simulink model "radar_lidar_road_curve"  (R2021b)
settings: Solver=FixedStepDiscrete  StartTime=0.0  StopTime=10.0  RelTol=1e-3
model workspace (MAT data in the model file):
  firstWarning = 1
  originalScenarioChecksum = '173E6664BED95618E8BCACADB1E8F97C'
libraries: drivingscenarioandsensors x3
settings Model: Creator=ghisl  LastModifiedBy=ghisl

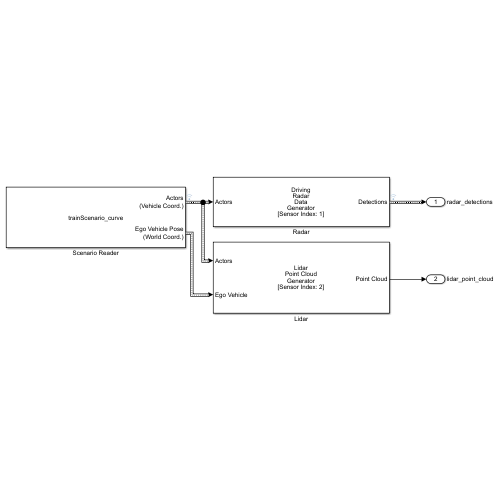
[thumbnail: Simulink's stored preview of the top-level diagram]
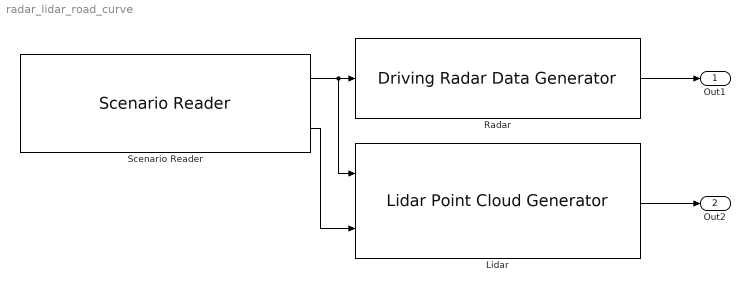
== system radar_lidar_road_curve ==
  Lidar : drivingscenarioandsensors/Lidar Point Cloud Generator  SensorIndex=2  UpdateInterval=0.1  SensorLocation=[0.05 0]  Height=1.6  Yaw=0  Pitch=0  Roll=0  DetectionCoordinates=Ego Cartesian  HasEgoVehicle=on  EgoVehicleActorID=2  HasRoadsInputPort=on  ActorProfilesSource=From Scenario Reader block  ActorProfilesVariableName=actor_profiles  MaxRange=120  RangeAccuracy=0.002  AzimuthResolution=0.16  ElevationResolution=1.25  AzimuthLimits=[-180 180]  ElevationLimits=[-20 20]  HasNoise=on
      settings: SourceProductBaseCode=DR
  Radar : drivingscenarioandsensors/Driving Radar Data Generator  SensorIndex=1  UpdateRate=10  MountingLocation=[1 0 0.2]  MountingAngles=[0 0 0]  HasElevation=off  HasRangeRate=on  HasNoise=on  HasFalseAlarms=on  HasOcclusion=on  MaxNumReportsSource=Property  MaxNumReports=50  TargetReportFormat=Detections  DetectionCoordinates=Body  TrackCoordinates=Body  BusNameSource=Auto  BusName=BusDrivingRadarDataGenerator  AzimuthResolution=4  ElevationResolution=5  RangeResolution=2.5  RangeRateResolution=0.5  AzimuthBiasFraction=0.1  ElevationBiasFraction=0.1  RangeBiasFraction=0.05  RangeRateBiasFraction=0.05  FieldOfView=[20 5]  RangeLimits=[0 100]  RangeRateLimits=[-100 100]  DetectionProbability=0.9  FalseAlarmRate=1e-06  ReferenceRange=100  ReferenceRCS=0  CenterFrequency=77000000000  FilterInitializationFcn=initcvekf  ConfirmationThreshold=[2 3]  DeletionThreshold=[5 5]  InitialSeedSource=Repeatable  InitialSeed=0  UsedSeed=0  ProfilesSource=Parameters  ProfilesParameters=driving.internal.ActorProfilesRadarParameters  ProfilesExpression=[struct('ActorID',1,'ClassID',7,'Length',20,'Width',2.8,'Height',4,'OriginOffset',[-9 0 0],'MeshVertices',[19 -1.4 4;19 1.4 4;-1 1.4 4;-1 -1.4 4;19 -1.4 0;19 1.4 0;-1 1.4 0;-1 -1.4 0],'MeshFaces',[6 2 1;1 5 6;8 4 3;3 7 8;6 7 3;3 2 6;5 1 4;4 8 5;4 1 2;2 3 4;7 6 5;5 8 7],'RCSPattern',[10 10;10 10],'RCSAzimuthAngles',[-180 180],'RCSElevationAngles',[-90 90]); struct('ActorID',2,'ClassID',8,'Length',2,'Width',0.6,'Height',1,'OriginOffset',[0 0 0],'MeshVertices',[1 0.3 0.612456747404844;1 -0.3 0.612456747404844;1 -0.3 0.224913494809689;1 0.3 0.224913494809689;1 0.3 0.612456747404844;0.5 0.3 0.709342560553633;0.5 -0.3 0.709342560553633;1 -0.3 0.612456747404844;0.2 0.24 1;-0.4 0.24 1;-0.4 -0.24 1;0.2 -0.24 1;-0.7 0.3 0.709342560553633;-1 0.3 0.612456747404844;-1 -0.3 0.612456747404844;-0.7 -0.3 0.709342560553633;1 0.3 0.612456747404844;1 0.3 0.224913494809689;0.5 0.3 0.224913494809689;0.5 0.3 0.709342560553633;0.5 0.3 0.709342560553633;0.5 0.3 0.224913494809689;-0.7 0.3 0.224913494809689;-0.7 0.3 0.709342560553633;-0.7 0.3 0.709342560553633;-0.7 0.3 0.224913494809689;-1 0.3 0.253979238754325;-1 0.3 0.612456747404844;0.5 0.3 0.709342560553633;-0.7 0.3 0.709342560553633;-0.4 0.24 1;0.2 0.24 1;1 -0.3 0.612456747404844;1 -0.3 0.224913494809689;0.5 -0.3 0.224913494809689;0.5 -0.3 0.709342560553633;0.5 -0.3 0.709342560553633;0.5 -0.3 0.224913494809689;-0.7 -0.3 0.224913494809689;-0.7 -0.3 0.709342560553633;-0.7 -0.3 0.709342560553633;-0.7 -0.3 0.224913494809689;-1 -0.3 0.253979238754325;-1 -0.3 0.612456747404844;0.5 -0.3 0.709342560553633;-0.7 -0.3 0.709342560553633;-0.4 -0.24 1;0.2 -0.24 1;-0.7 0.3 0.709342560553633;-0.7 -0.3 0.709342560553633;-0.4 -0.24 1;-0.4 0.24 1;0.5 -0.3 0.709342560553633;0.2 -0.24 1;0.2 0.24 1;0.5 0.3 0.709342560553633;-1 0.3 0.612456747404844;-1 0.3 0.253979238754325;-1 -0.3 0.253979238754325;-1 -0.3 0.612456747404844;1 0.3 0.224913494809689;1 -0.3 0.224913494809689;-0.7 -0.3 0.224913494809689;-0.7 0.3 0.224913494809689;-0.7 0.3 0.224913494809689;-1 0.3 0.253979238754325;-1 -0.3 0.253979238754325;-0.7 -0.3 0.224913494809689;-0.574468085106383 -0.21 0;-0.574468085106383 -0.29 0;-0.493178635321254 -0.21 0.042954655244389;-0.493178635321254 -0.29 0.042954655244389;-0.442938992427266 -0.21 0.155411402649233;-0.442938992427266 -0.29 0.155411402649233;-0.442938992427266 -0.21 0.294415586970144;-0.442938992427266 -0.29 0.294415586970144;-0.493178635321254 -0.21 0.406872334374988;-0.493178635321254 -0.29 0.406872334374988;-0.574468085106383 -0.21 0.449826989619377;-0.574468085106383 -0.29 0.449826989619377;-0.655757534891512 -0.21 0.406872334374988;-0.655757534891512 -0.29 0.406872334374988;-0.7059971777855 -0.21 0.294415586970144;-0.7059971777855 -0.29 0.294415586970144;-0.7059971777855 -0.21 0.155411402649233;-0.7059971777855 -0.29 0.155411402649233;-0.655757534891512 -0.21 0.042954655244389;-0.655757534891512 -0.29 0.042954655244389;-0.574468085106383 -0.21 0;-0.574468085106383 -0.29 0;-0.574468085106383 -0.21 0;-0.493178635321254 -0.21 0.042954655244389;-0.442938992427266 -0.21 0.155411402649233;-0.442938992427266 -0.21 0.294415586970144;-0.493178635321254 -0.21 0.406872334374988;-0.574468085106383 -0.21 0.449826989619377;-0.655757534891512 -0.21 0.406872334374988;-0.7059971777855 -0.21 0.294415586970144;-0.7059971777855 -0.21 0.155411402649233;-0.655757534891512 -0.21 0.042954655244389;-0.574468085106383 -0.29 0;-0.493178635321254 -0.29 0.042954655244389;-0.442938992427266 -0.29 0.155411402649233;-0.442938992427266 -0.29 0.294415586970144;-0.493178635321254 -0.29 0.406872334374988;-0.574468085106383 -0.29 0.449826989619377;-0.655757534891512 -0.29 0.406872334374988;-0.7059971777855 -0.29 0.294415586970144;-0.7059971777855 -0.29 0.155411402649233;-0.655757534891512 -0.29 0.042954655244389;-0.574468085106383 0.29 0;-0.574468085106383 0.21 0;-0.493178635321254 0.29 0.042954655244389;-0.493178635321254 0.21 0.042954655244389;-0.442938992427266 0.29 0.155411402649233;-0.442938992427266 0.21 0.155411402649233;-0.442938992427266 0.29 0.294415586970144;-0.442938992427266 0.21 0.294415586970144;-0.493178635321254 0.29 0.406872334374988;-0.493178635321254 0.21 0.406872334374988;-0.574468085106383 0.29 0.449826989619377;-0.574468085106383 0.21 0.449826989619377;-0.655757534891512 0.29 0.406872334374988;-0.655757534891512 0.21 0.406872334374988;-0.7059971777855 0.29 0.294415586970144;-0.7059971777855 0.21 0.294415586970144;-0.7059971777855 0.29 0.155411402649233;-0.7059971777855 ...(+4253 chars)],'MeshFaces',[1 2 3;3 4 1;5 6 7;7 8 5;9 10 11;11 12 9;13 14 15;15 16 13;17 18 19;19 20 17;21 22 23;23 24 21;25 26 27;27 28 25;29 30 31;31 32 29;33 34 35;35 36 33;37 38 39;39 40 37;41 42 43;43 44 41;45 46 47;47 48 45;49 50 51;51 52 49;53 54 55;55 56 53;57 58 59;59 60 57;61 62 63;63 64 61;65 66 67;67 68 65;69 71 72;72 70 69;71 73 74;74 72 71;73 75 76;76 74 73;75 77 78;78 76 75;77 79 80;80 78 77;79 81 82;82 80 79;81 83 84;84 82 81;83 85 86;86 84 83;85 87 88;88 86 85;87 89 90;90 88 87;91 92 93;91 93 94;91 94 95;91 95 96;91 96 97;91 97 98;91 98 99;91 99 100;101 102 103;101 103 104;101 104 105;101 105 106;101 106 107;101 107 108;101 108 109;101 109 110;111 113 114;114 112 111;113 115 116;116 114 113;115 117 118;118 116 115;117 119 120;120 118 117;119 121 122;122 120 119;121 123 124;124 122 121;123 125 126;126 124 123;125 127 128;128 126 125;127 129 130;130 128 127;129 131 132;132 130 129;133 134 135;133 135 136;133 136 137;133 137 138;133 138 139;133 139 140;133 140 141;133 141 142;143 144 145;143 145 146;143 146 147;143 147 148;143 148 149;143 149 150;143 150 151;143 151 152;153 155 156;156 154 153;155 157 158;158 156 155;157 159 160;160 158 157;159 161 162;162 160 159;161 163 164;164 162 161;163 165 166;166 164 163;165 167 168;168 166 165;167 169 170;170 168 167;169 171 172;172 170 169;171 173 174;174 172 171;175 176 177;175 177 178;175 178 179;175 179 180;175 180 181;175 181 182;175 182 183;175 183 184;185 186 187;185 187 188;185 188 189;185 189 190;185 190 191;185 191 192;185 192 193;185 193 194;195 197 198;198 196 195;197 199 200;200 198 197;199 201 202;202 200 199;201 203 204;204 202 201;203 205 206;206 204 203;205 207 208;208 206 205;207 209 210;210 208 207;209 211 212;212 210 209;211 213 214;214 212 211;213 215 216;216 214 213;217 218 219;217 219 220;217 220 221;217 221 222;217 222 223;217 223 224;217 224 225;217 225 226;227 228 229;227 229 230;227 230 231;227 231 232;227 232 233;227 233 234;227 234 235;227 235 236],'RCSPattern',[10 10;10 10],'RCSAzimuthAngles',[-180 180],'RCSElevationAngles',[-90 90])]
      settings: SourceProductBaseCode=DR
  Scenario Reader : drivingscenarioandsensors/Scenario Reader  ScenarioSource=From file  ScenarioFileName=G:\My Drive\UniBG\CORSI\Laurea Magistrale\2021_2022 - Magistrale Secondo Anno\secondo_semestre\Tirocinio Formativo\tirocinio_PRSE\matlab_stuff\simulink_simulations\trainScenario_curve.mat  ScenarioVariableName=scenario  OutputCoordinateSystem=Vehicle coordinates  EgoVehicleSource=Scenario  EgoVehicleActorID=1  OrientVehiclesOnRoad=off  OutputEgoVehiclePose=on  OutputEgoVehicleState=off  SampleTime=0.1  LaneBoundaryOutput=None  LaneBoundaryDistance=0:0.5:9.5  LaneBoundaryLocation=Center of lane markings  BusNameSource=Auto  BusName=BusActors  BusNumActorsSource=Scenario  BusNumActors=100  BusName2Source=Auto  BusName2=BusLaneBoundaries  BusNumLaneBoundariesSource=Scenario  BusNumLaneBoundaries=10  BusName3Source=Auto  BusName3=BusEgoActor  BusName4Source=Auto  BusName4=BusEgoState  ShowCoordinateLabels=on  SimulateUsing=Interpreted execution
  Out1 : Outport  SignalName=radar_detections
  Out2 : Outport  Port=2  SignalName=lidar_point_cloud
  wires:
  Scenario Reader/1 -> Radar/1, Lidar/1
  Scenario Reader/2 -> Lidar/2
  Radar/1 -> Out1/1
  Lidar/1 -> Out2/1
